simulink model "shelvingEqualiser"  (Simulink 6.6)
settings: Solver=ode45  StartTime=0.0  StopTime=inf  RelTol=1e-3
libraries: dspsrcs4 x1, simulink_extras x1
settings Model: Creator=student  LastModifiedBy=student

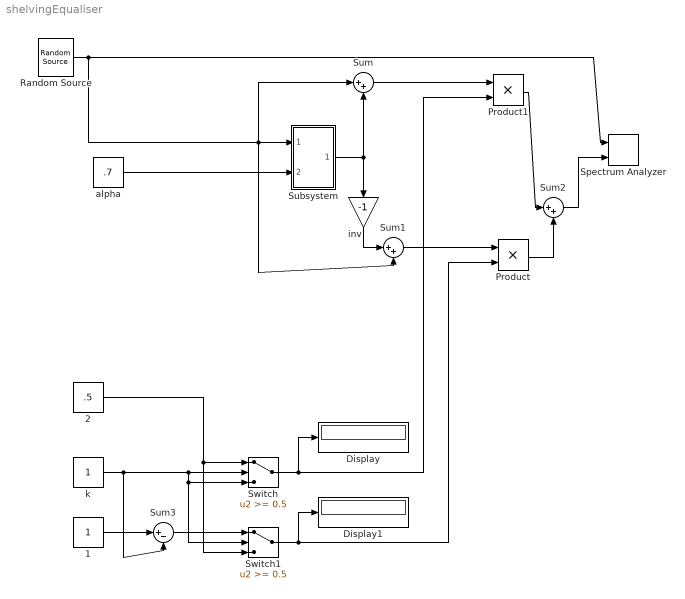
== system shelvingEqualiser ==
  1 : Constant
  2 : Constant  Value=.5
  Display : Display
  Display1 : Display
  Product : Product  RndMeth=Zero
  Product1 : Product  RndMeth=Zero
  Random Source : dspsrcs4/Random Source  SrcType=Gaussian  NormMethod=Ziggurat  CltLength=12  MinVal=-1  MaxVal=1  MeanVal=0  VarVal=1  RepMode=Not repeatable  rawSeed=1  IsInherit=off  SampMode=Discrete  SampTime=1  SampFrame=1  DataType=Double  OutComplex=Real
  Spectrum Analyzer : simulink_extras/Additional Sinks/Spectrum Analyzer  SystemSampleTime=-1  npts=256  fftpts=256  HowOften=64  sampleT=1
  Subsystem : Subsystem
  Sum : Sum  Inputs=|++
  Sum1 : Sum  Inputs=|++
  Sum2 : Sum  Inputs=|++
  Sum3 : Sum  Inputs=|+-
  Switch : Switch  Threshold=0.5
  Switch1 : Switch  Threshold=0.5
  alpha : Constant  Value=.7
  inv : Gain  Orientation=down  Gain=-1
  k : Constant
  wires:
  Random Source/1 -> Spectrum Analyzer/1, Subsystem/1(In1), Sum/1, Sum1/2
  Subsystem/1(Out1) -> inv/1, Sum/2
  alpha/1 -> Subsystem/2(alpha)
  Sum/1 -> Product1/1
  Sum1/1 -> Product/1
  Product/1 -> Sum2/2
  Product1/1 -> Sum2/1
  Sum2/1 -> Spectrum Analyzer/2
  inv/1 -> Sum1/1
  k/1 -> Switch/2, Switch1/2, Switch/3, Sum3/2
  Switch/1 -> Product1/2, Display/1
  Switch1/1 -> Product/2, Display1/1
  1/1 -> Sum3/1
  2/1 -> Switch/1, Switch1/3
  Sum3/1 -> Switch1/1

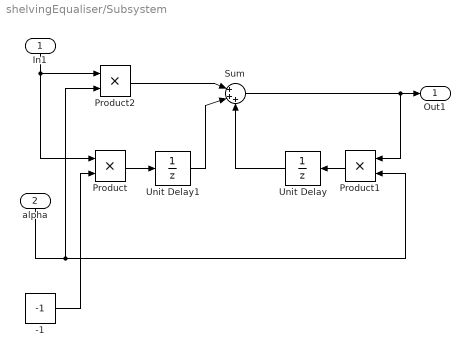
== system shelvingEqualiser/Subsystem ==
  In1 : Inport  Orientation=down
  alpha : Inport  Orientation=down  Port=2
  -1 : Constant  Value=-1
  Product : Product  RndMeth=Zero
  Product1 : Product  Orientation=left  RndMeth=Zero
  Product2 : Product  RndMeth=Zero
  Sum : Sum  Inputs=|+++
  Unit Delay : UnitDelay  Orientation=left
  Unit Delay1 : UnitDelay
  Out1 : Outport
  wires:
  Product/1 -> Unit Delay1/1
  Product1/1 -> Unit Delay/1
  Unit Delay1/1 -> Sum/2
  Unit Delay/1 -> Sum/3
  alpha/1 -> Product1/2, Product2/2
  Sum/1 -> Product1/1, Out1/1
  Product2/1 -> Sum/1
  -1/1 -> Product/2
  In1/1 -> Product/1, Product2/1
